simulink model "FinalBidirectionalACDC"  (R2020b)
settings: Solver=VariableStepAuto  StartTime=0.0  StopTime=10.0  RelTol=1e-3
libraries: powerlib x46, powerlib_meascontrol x13, pid_lib x4, eePowerMeasurement x1, simulink x1
settings Model: Creator=Matthew  LastModifiedBy=Matthew

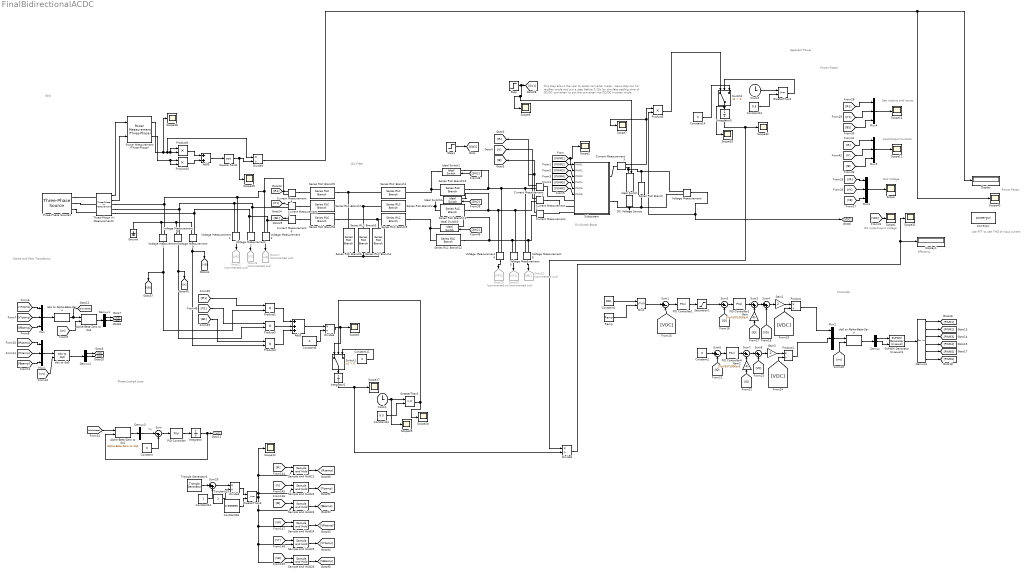
== system FinalBidirectionalACDC ==
  note: Power Factor
  note: Use FFT to see THD of input current
  note: Efficiency
  note: This step allows the user to select converter mode -
      |  leave step low for rectifier mode and put a step before 0.15s
      | (to simulate settling time of DC/DC converter) to put the converter
      | into DC/DC inverter mode.
  note: DC output/input voltage
  note: Power Factor
  note: Apparent Power
  note: Grid
  note: Vq
  note: Phase-Locked
      | Loop
  note: Six-Switch
      | Boost
  note: Grid Voltage
  note: LCL Filter
  note: See outputs and inputs
  note: Input/Output Currents
  note: Clarke and Park
      | Transforms
  note: Controller
  Add3 : Sum  Inputs=+++
  Add6 : Sum
  Alpha-Beta-Zero to dq0 : powerlib_meascontrol/Transformations/Alpha-Beta-Zero to dq0  Alignment=90 degrees behind phase A axis
  Alpha-Beta-Zero to dq1 : powerlib_meascontrol/Transformations/Alpha-Beta-Zero to dq0  Alignment=90 degrees behind phase A axis
  Clock1 : Clock
  Clock2 : Clock
  Constant{,2,11,14} (4 alike) : Constant  Value=0
  Constant1 : Constant  Value=800
  Constant12 : Constant  Value=0.5
  Constant13 : Constant  Value=0.5
  Constant24 : Constant
  Constant25 : Constant  Value=2
  Constant26 : Constant  Value=0.999999
  Constant6 : Constant  Value=-1
  Current Measurement{,1..6} (7 alike) : powerlib/Measurements/Current Measurement  PhasorSimulation=off  OutputType=Complex  PSBequivalent=0
  DC Voltage Source : powerlib/Electrical Sources/DC Voltage Source  Amplitude=800  Measurements=None
  Demux{,1..3} (4 alike) : Demux  Outputs=3
  Demux4 : Demux  Outputs=6
  Display : Display
  Display1 : Display
  Divide{3,6,8..9} (4 alike) : Product  Inputs=*/
  Gain : Gain  Gain=2*pi*50*1000e-6
  Gain1 : Gain  Gain=2
  Gain2 : Gain  Gain=2*pi*50*1000e-6
  Gain3 : Gain  Gain=2
  Goto22 : Goto  Commented=on  GotoTag=VR
  Goto26 : Goto  Commented=on  GotoTag=VY
  Goto27 : Goto  Commented=on  GotoTag=VB
  Goto29 : Goto  Commented=on  GotoTag=VR1
  Goto30 : Goto  Commented=on  GotoTag=VY1
  Goto33 : Goto  Commented=on  GotoTag=VB1
  GreaterThan1 : RelationalOperator  OutDataTypeStr=boolean  RndMeth=Simplest
  GreaterThan2 : RelationalOperator  OutDataTypeStr=boolean  RndMeth=Simplest
  GreaterThan3 : RelationalOperator  OutDataTypeStr=boolean  RndMeth=Simplest
  Ground : powerlib/Elements/Ground  LConnTagsString=a
  Ideal Switch : powerlib/Power Electronics/Ideal Switch  Ron=1e-15  Lon=0  IC=0  Rs=inf  Cs=inf  Measurements=off
  Ideal Switch1 : powerlib/Power Electronics/Ideal Switch  Ron=1e-9  Lon=0  IC=0  Rs=inf  Cs=inf  Measurements=off
  Ideal Switch2 : powerlib/Power Electronics/Ideal Switch  Ron=1e-9  Lon=0  IC=0  Rs=inf  Cs=inf  Measurements=off
  Ideal Switch3 : powerlib/Power Electronics/Ideal Switch  Ron=1e-9  Lon=0  IC=0  Rs=inf  Cs=inf  Measurements=off
  Integrator : Integrator
  Integrator2 : Integrator
  Integrator3 : Integrator
  Min1 : MinMax  Inputs=2
  Mux{,1..5} (6 alike) : Mux  Inputs=3
  PID Controller : pid_lib/PID Controller  Controller=PI  Form=Parallel  TimeDomain=Continuous-time  UseExternalTs=off  SampleTime=-1  IntegratorMethod=Forward Euler  FilterMethod=Forward Euler  ControllerParametersSource=internal  P=10  I=100000  D=0  UseFilter=on  N=100  TunerSelectOption=Transfer Function Based (PID Tuner App)  InitialConditionSource=internal  InitialConditionForIntegrator=0  InitialConditionForFilter=0  DifferentiatorICPrevScaledInput=0  ExternalReset=none  TrackingMode=off  Kt=1  LimitOutput=off  SatLimitsSource=internal  UpperSaturationLimit=inf  LowerSaturationLimit=-inf  LinearizeAsGain=on  AntiWindupMode=none  Kb=1  POutMin=[]  POutMax=[]  IOutMin=[]  IOutMax=[]  DOutMin=[]  DOutMax=[]  NOutMin=[]  NOutMax=[]  SumOutMin=[]  SumOutMax=[]  SaturationOutMin=[]  SaturationOutMax=[]  PParamMin=[]  PParamMax=[]  IParamMin=[]  IParamMax=[]  DParamMin=[]  DParamMax=[]  NParamMin=[]  NParamMax=[]  KbParamMin=[]  KbParamMax=[]  KtParamMin=[]  KtParamMax=[]  KbOutMin=[]  KbOutMax=[]  KtOutMin=[]  KtOutMax=[]  IntegratorOutMin=[]  IntegratorOutMax=[]  FilterOutMin=[]  FilterOutMax=[]  SumI1OutMin=[]  SumI1OutMax=[]  SumI2OutMin=[]  SumI2OutMax=[]  SumI3OutMin=[]  SumI3OutMax=[]  SumI4OutMin=[]  SumI4OutMax=[]  SumDOutMin=[]  SumDOutMax=[]  DifferentiatorOutMin=[]  DifferentiatorOutMax=[]  FilterDiffOutCoefMin=[]  FilterDiffOutCoefMax=[]  ReciprocalOutMin=[]  ReciprocalOutMax=[]  SumDenOutMin=[]  SumDenOutMax=[]  SumNumOutMin=[]  SumNumOutMax=[]  DivideOutMin=[]  DivideOutMax=[]  UdiffTsProdOutMin=[]  UdiffTsProdOutMax=[]  NTsProdOutMin=[]  NTsProdOutMax=[]  UintegralTsProdOutMin=[]  UintegralTsProdOutMax=[]  UngainTsProdOutMin=[]  UngainTsProdOutMax=[]  IntegratorContinuousStateAttributes=''  IntegratorStateMustResolveToSignalObject=off  IntegratorRTWStateStorageClass=Auto  FilterContinuousStateAttributes=''  FilterStateMustResolveToSignalObject=off  FilterRTWStateStorageClass=Auto  ParallelPVariant=InternalParameters  IdealPVariant=Disabled  IVariant=InternalParameters  DVariant=Disabled  IntegratorVariant=Continuous  SatVariant=Disabled  AWVariant=Passthrough  PCopyVariant=Disabled  TRVariant=Disabled  FdbkBlocksVariant=Forward  IdealPFdbkVariant=Disabled  SatFdbkVariant=Disabled  DerivativeFilterVariant=Disabled  NVariant=Disabled  NCopyVariant=Disabled_SignalSpec  FilterICVariant=Disabled  IntegratorICVariant=InternalICs  ExternalResetVariant=Disabled  TRSumVariant=Passthrough  SumFdbkVariant=Disabled  SumVariant=Sum_PI  TsampFilterVariant=InternalTs  TsampNgainVariant=Passthrough  TsampIntegralVariant=Passthrough  ExternalSaturationOutDataTypeStr=Inherit: Same as second input
  PID Controller1 : pid_lib/PID Controller  Controller=PI  Form=Parallel  TimeDomain=Continuous-time  UseExternalTs=off  SampleTime=-1  IntegratorMethod=Forward Euler  FilterMethod=Forward Euler  ControllerParametersSource=internal  P=0.15  I=22  D=0  UseFilter=on  N=100  TunerSelectOption=Transfer Function Based (PID Tuner App)  InitialConditionSource=internal  InitialConditionForIntegrator=0  InitialConditionForFilter=0  DifferentiatorICPrevScaledInput=0  ExternalReset=none  TrackingMode=off  Kt=1  LimitOutput=off  SatLimitsSource=internal  UpperSaturationLimit=inf  LowerSaturationLimit=-inf  LinearizeAsGain=on  AntiWindupMode=none  Kb=1  POutMin=[]  POutMax=[]  IOutMin=[]  IOutMax=[]  DOutMin=[]  DOutMax=[]  NOutMin=[]  NOutMax=[]  SumOutMin=[]  SumOutMax=[]  SaturationOutMin=[]  SaturationOutMax=[]  PParamMin=[]  PParamMax=[]  IParamMin=[]  IParamMax=[]  DParamMin=[]  DParamMax=[]  NParamMin=[]  NParamMax=[]  KbParamMin=[]  KbParamMax=[]  KtParamMin=[]  KtParamMax=[]  KbOutMin=[]  KbOutMax=[]  KtOutMin=[]  KtOutMax=[]  IntegratorOutMin=[]  IntegratorOutMax=[]  FilterOutMin=[]  FilterOutMax=[]  SumI1OutMin=[]  SumI1OutMax=[]  SumI2OutMin=[]  SumI2OutMax=[]  SumI3OutMin=[]  SumI3OutMax=[]  SumI4OutMin=[]  SumI4OutMax=[]  SumDOutMin=[]  SumDOutMax=[]  DifferentiatorOutMin=[]  DifferentiatorOutMax=[]  FilterDiffOutCoefMin=[]  FilterDiffOutCoefMax=[]  ReciprocalOutMin=[]  ReciprocalOutMax=[]  SumDenOutMin=[]  SumDenOutMax=[]  SumNumOutMin=[]  SumNumOutMax=[]  DivideOutMin=[]  DivideOutMax=[]  UdiffTsProdOutMin=[]  UdiffTsProdOutMax=[]  NTsProdOutMin=[]  NTsProdOutMax=[]  UintegralTsProdOutMin=[]  UintegralTsProdOutMax=[]  UngainTsProdOutMin=[]  UngainTsProdOutMax=[]  IntegratorContinuousStateAttributes=''  IntegratorStateMustResolveToSignalObject=off  IntegratorRTWStateStorageClass=Auto  FilterContinuousStateAttributes=''  FilterStateMustResolveToSignalObject=off  FilterRTWStateStorageClass=Auto  ParallelPVariant=InternalParameters  IdealPVariant=Disabled  IVariant=InternalParameters  DVariant=Disabled  IntegratorVariant=Continuous  SatVariant=Disabled  AWVariant=Passthrough  PCopyVariant=Disabled  TRVariant=Disabled  FdbkBlocksVariant=Forward  IdealPFdbkVariant=Disabled  SatFdbkVariant=Disabled  DerivativeFilterVariant=Disabled  NVariant=Disabled  NCopyVariant=Disabled_SignalSpec  FilterICVariant=Disabled  IntegratorICVariant=InternalICs  ExternalResetVariant=Disabled  TRSumVariant=Passthrough  SumFdbkVariant=Disabled  SumVariant=Sum_PI  TsampFilterVariant=InternalTs  TsampNgainVariant=Passthrough  TsampIntegralVariant=Passthrough  ExternalSaturationOutDataTypeStr=Inherit: Same as second input
  PID Controller2 : pid_lib/PID Controller  Controller=PI  Form=Parallel  TimeDomain=Continuous-time  UseExternalTs=off  SampleTime=-1  IntegratorMethod=Forward Euler  FilterMethod=Forward Euler  ControllerParametersSource=internal  P=25  I=500  D=0  UseFilter=on  N=100  TunerSelectOption=Transfer Function Based (PID Tuner App)  InitialConditionSource=internal  InitialConditionForIntegrator=0  InitialConditionForFilter=0  DifferentiatorICPrevScaledInput=0  ExternalReset=none  TrackingMode=off  Kt=1  LimitOutput=off  SatLimitsSource=internal  UpperSaturationLimit=inf  LowerSaturationLimit=-inf  LinearizeAsGain=on  AntiWindupMode=none  Kb=1  POutMin=[]  POutMax=[]  IOutMin=[]  IOutMax=[]  DOutMin=[]  DOutMax=[]  NOutMin=[]  NOutMax=[]  SumOutMin=[]  SumOutMax=[]  SaturationOutMin=[]  SaturationOutMax=[]  PParamMin=[]  PParamMax=[]  IParamMin=[]  IParamMax=[]  DParamMin=[]  DParamMax=[]  NParamMin=[]  NParamMax=[]  KbParamMin=[]  KbParamMax=[]  KtParamMin=[]  KtParamMax=[]  KbOutMin=[]  KbOutMax=[]  KtOutMin=[]  KtOutMax=[]  IntegratorOutMin=[]  IntegratorOutMax=[]  FilterOutMin=[]  FilterOutMax=[]  SumI1OutMin=[]  SumI1OutMax=[]  SumI2OutMin=[]  SumI2OutMax=[]  SumI3OutMin=[]  SumI3OutMax=[]  SumI4OutMin=[]  SumI4OutMax=[]  SumDOutMin=[]  SumDOutMax=[]  DifferentiatorOutMin=[]  DifferentiatorOutMax=[]  FilterDiffOutCoefMin=[]  FilterDiffOutCoefMax=[]  ReciprocalOutMin=[]  ReciprocalOutMax=[]  SumDenOutMin=[]  SumDenOutMax=[]  SumNumOutMin=[]  SumNumOutMax=[]  DivideOutMin=[]  DivideOutMax=[]  UdiffTsProdOutMin=[]  UdiffTsProdOutMax=[]  NTsProdOutMin=[]  NTsProdOutMax=[]  UintegralTsProdOutMin=[]  UintegralTsProdOutMax=[]  UngainTsProdOutMin=[]  UngainTsProdOutMax=[]  IntegratorContinuousStateAttributes=''  IntegratorStateMustResolveToSignalObject=off  IntegratorRTWStateStorageClass=Auto  FilterContinuousStateAttributes=''  FilterStateMustResolveToSignalObject=off  FilterRTWStateStorageClass=Auto  ParallelPVariant=InternalParameters  IdealPVariant=Disabled  IVariant=InternalParameters  DVariant=Disabled  IntegratorVariant=Continuous  SatVariant=Disabled  AWVariant=Passthrough  PCopyVariant=Disabled  TRVariant=Disabled  FdbkBlocksVariant=Forward  IdealPFdbkVariant=Disabled  SatFdbkVariant=Disabled  DerivativeFilterVariant=Disabled  NVariant=Disabled  NCopyVariant=Disabled_SignalSpec  FilterICVariant=Disabled  IntegratorICVariant=InternalICs  ExternalResetVariant=Disabled  TRSumVariant=Passthrough  SumFdbkVariant=Disabled  SumVariant=Sum_PI  TsampFilterVariant=InternalTs  TsampNgainVariant=Passthrough  TsampIntegralVariant=Passthrough  ExternalSaturationOutDataTypeStr=Inherit: Same as second input
  PID Controller4 : pid_lib/PID Controller  Controller=PI  Form=Parallel  TimeDomain=Continuous-time  UseExternalTs=off  SampleTime=-1  IntegratorMethod=Forward Euler  FilterMethod=Forward Euler  ControllerParametersSource=internal  P=25  I=500  D=0  UseFilter=on  N=100  TunerSelectOption=Transfer Function Based (PID Tuner App)  InitialConditionSource=internal  InitialConditionForIntegrator=0  InitialConditionForFilter=0  DifferentiatorICPrevScaledInput=0  ExternalReset=none  TrackingMode=off  Kt=1  LimitOutput=off  SatLimitsSource=internal  UpperSaturationLimit=inf  LowerSaturationLimit=-inf  LinearizeAsGain=on  AntiWindupMode=none  Kb=1  POutMin=[]  POutMax=[]  IOutMin=[]  IOutMax=[]  DOutMin=[]  DOutMax=[]  NOutMin=[]  NOutMax=[]  SumOutMin=[]  SumOutMax=[]  SaturationOutMin=[]  SaturationOutMax=[]  PParamMin=[]  PParamMax=[]  IParamMin=[]  IParamMax=[]  DParamMin=[]  DParamMax=[]  NParamMin=[]  NParamMax=[]  KbParamMin=[]  KbParamMax=[]  KtParamMin=[]  KtParamMax=[]  KbOutMin=[]  KbOutMax=[]  KtOutMin=[]  KtOutMax=[]  IntegratorOutMin=[]  IntegratorOutMax=[]  FilterOutMin=[]  FilterOutMax=[]  SumI1OutMin=[]  SumI1OutMax=[]  SumI2OutMin=[]  SumI2OutMax=[]  SumI3OutMin=[]  SumI3OutMax=[]  SumI4OutMin=[]  SumI4OutMax=[]  SumDOutMin=[]  SumDOutMax=[]  DifferentiatorOutMin=[]  DifferentiatorOutMax=[]  FilterDiffOutCoefMin=[]  FilterDiffOutCoefMax=[]  ReciprocalOutMin=[]  ReciprocalOutMax=[]  SumDenOutMin=[]  SumDenOutMax=[]  SumNumOutMin=[]  SumNumOutMax=[]  DivideOutMin=[]  DivideOutMax=[]  UdiffTsProdOutMin=[]  UdiffTsProdOutMax=[]  NTsProdOutMin=[]  NTsProdOutMax=[]  UintegralTsProdOutMin=[]  UintegralTsProdOutMax=[]  UngainTsProdOutMin=[]  UngainTsProdOutMax=[]  IntegratorContinuousStateAttributes=''  IntegratorStateMustResolveToSignalObject=off  IntegratorRTWStateStorageClass=Auto  FilterContinuousStateAttributes=''  FilterStateMustResolveToSignalObject=off  FilterRTWStateStorageClass=Auto  ParallelPVariant=InternalParameters  IdealPVariant=Disabled  IVariant=InternalParameters  DVariant=Disabled  IntegratorVariant=Continuous  SatVariant=Disabled  AWVariant=Passthrough  PCopyVariant=Disabled  TRVariant=Disabled  FdbkBlocksVariant=Forward  IdealPFdbkVariant=Disabled  SatFdbkVariant=Disabled  DerivativeFilterVariant=Disabled  NVariant=Disabled  NCopyVariant=Disabled_SignalSpec  FilterICVariant=Disabled  IntegratorICVariant=InternalICs  ExternalResetVariant=Disabled  TRSumVariant=Passthrough  SumFdbkVariant=Disabled  SumVariant=Sum_PI  TsampFilterVariant=InternalTs  TsampNgainVariant=Passthrough  TsampIntegralVariant=Passthrough  ExternalSaturationOutDataTypeStr=Inherit: Same as second input
  Power Measurement (Three-Phase) : eePowerMeasurement/Power Measurement (Three-Phase)  LabelModeActiveChoice=Continuous  F=50  K=[1]  Seq=Positive  Ts=0
      settings: SourceProductBaseCode=PS
  Product : Product  Inputs=*/
  Product1 : Product  Inputs=*/
  Product{2..5,9..10} (6 alike) : Product
  Ramp : simulink/Sources/Ramp  slope=450  start=0  InitialOutput=700
  SVPWM Generator (2-Level)1 : powerlib_meascontrol/Pulse & Signal Generators/SVPWM Generator (2-Level)  InputType=alpha-beta components  SwitchingPattern=Pattern #2  Fc=100e3  ParUref=[0.8 -30 50]  Ts=0
      settings: SourceProductBaseCode=PS
  Sample and Hold{21..26} (6 alike) : powerlib_meascontrol/Additional Components/Sample and Hold  ic=0  Ts=0
      settings: SourceProductBaseCode=PS
  Saturation1 : Saturate  UpperLimit=450  LowerLimit=-240
  Scope{,1..2,5,7,9,11..12,14,17,28..29,31..33,40,48..49} (18 alike) : Scope
  Series RLC Branch : powerlib/Elements/Series RLC Branch  LConnTagsString=__new0  RConnTagsString=__new0  BranchType=R  Resistance=6.4  Inductance=1e-3  SetiL0=off  InitialCurrent=0  Capacitance=1e-6  Setx0=off  InitialVoltage=0  Measurements=None
  Series RLC Branch{1..2,5,7..9} (6 alike) : powerlib/Elements/Series RLC Branch  LConnTagsString=__new0  RConnTagsString=__new0  BranchType=RL  Resistance=13.5e-3  Inductance=150e-6  SetiL0=off  InitialCurrent=0  Capacitance=0  Setx0=off  InitialVoltage=0  Measurements=None
  Series RLC Branch10 : powerlib/Elements/Series RLC Branch  LConnTagsString=__new0  RConnTagsString=__new0  BranchType=R  Resistance=1  Inductance=1e-3  SetiL0=off  InitialCurrent=0  Capacitance=1e-6  Setx0=off  InitialVoltage=0  Measurements=None
  Series RLC Branch11 : powerlib/Elements/Series RLC Branch  LConnTagsString=__new0  RConnTagsString=__new0  BranchType=R  Resistance=1  Inductance=1e-3  SetiL0=off  InitialCurrent=0  Capacitance=1e-6  Setx0=off  InitialVoltage=0  Measurements=None
  Series RLC Branch12 : powerlib/Elements/Series RLC Branch  LConnTagsString=__new0  RConnTagsString=__new0  BranchType=R  Resistance=1  Inductance=1e-3  SetiL0=off  InitialCurrent=0  Capacitance=1e-6  Setx0=off  InitialVoltage=0  Measurements=None
  Series RLC Branch3 : powerlib/Elements/Series RLC Branch  LConnTagsString=__new0  RConnTagsString=__new0  BranchType=RC  Resistance=10e-3  Inductance=1e-3  SetiL0=off  InitialCurrent=0  Capacitance=2e-5  Setx0=off  InitialVoltage=0  Measurements=None
  Series RLC Branch4 : powerlib/Elements/Series RLC Branch  LConnTagsString=__new0  RConnTagsString=__new0  BranchType=RC  Resistance=10e-3  Inductance=1e-3  SetiL0=off  InitialCurrent=0  Capacitance=2e-5  Setx0=off  InitialVoltage=0  Measurements=None
  Series RLC Branch6 : powerlib/Elements/Series RLC Branch  LConnTagsString=__new0  RConnTagsString=__new0  BranchType=RC  Resistance=10e-3  Inductance=1e-3  SetiL0=off  InitialCurrent=0  Capacitance=2e-5  Setx0=off  InitialVoltage=0  Measurements=None
  Square Root1 : Sqrt  SaturateOnIntegerOverflow=on
  Step : Step  Time=10  SampleTime=0
  Step1 : Step  Time=0.02  SampleTime=0
  Subsystem : Subsystem
  Sum : Sum  Inputs=|-+
  Sum{1..2,6..7} (4 alike) : Sum  Inputs=|+-
  Sum{3..4,8,29} (4 alike) : Sum  Inputs=|++
  Switch1 : Switch  Criteria=u2 > Threshold
  Switch2 : Switch  Criteria=u2 > Threshold
  Three-Phase V-I Measurement2 : powerlib/Measurements/Three-Phase V-I Measurement  VoltageMeasurement=phase-to-ground  SetLabelV=off  LabelV=Vabc  Vpu=off  VpuLL=off  CurrentMeasurement=yes  SetLabelI=off  LabelI=Iabc  Ipu=off  Pbase=100e6  Vbase=500e3  OutputType=Complex  PhasorSimulation=off  PSBequivalent=0
  Three-Phase Source1 : powerlib/Electrical Sources/Three-Phase Source  InternalConnection=Yg  VoltagePhases=off  Voltage=400  PhaseAngle=0  Voltage_phases=[25e3 25e3 25e3]/sqrt(3)  PhaseAngles_phases=[0 -120 +120]  Frequency=50  NonIdealSource=on  SpecifyImpedance=off  Resistance=0  Inductance=0  ShortCircuitLevel=100e6  BaseVoltage=400  XRratio=7  BusType=swing  Pref=10e3  Qref=0  Prefabc=[10e3, 10e3, 10e3]  Qrefabc=[0, 0, 0]  Qmin=-inf  Qmax=inf
  Triangle Generator3 : powerlib_meascontrol/Pulse & Signal Generators/Triangle Generator  Freq=100e3  Phase=180  Ts=0
  Voltage Measurement{,1..9} (10 alike) : powerlib/Measurements/Voltage Measurement  PhasorSimulation=off  OutputType=Complex  PSBequivalent=0
  abc to Alpha-Beta-Zero : powerlib_meascontrol/Transformations/abc to Alpha-Beta-Zero
  abc to dq0 : powerlib_meascontrol/Transformations/abc to dq0  Alignment=90 degrees behind phase A axis
  dq0 to Alpha-Beta-Zero : powerlib_meascontrol/Transformations/dq0 to Alpha-Beta-Zero  Alignment=90 degrees behind phase A axis
      settings: SourceProductBaseCode=PS
  powergui : powerlib/powergui  Priority=1  SimulationMode=Discrete  SampleTime=1e-6  frequency=60  Iterations=50  frequencyindice=0  Pbase=100e6  ErrMax=1e-4  UnitsV=kV  UnitsW=MW  buscounter=0  FunctionMessages=off  echomessages=off  EnableUseOfTLC=off  CurrentSourceSwitches=off  DisableSnubberDevices=off  DisableRonSwitches=off  DisableVfSwitches=off  DisplayEquations=off  AutomaticDiscreteSolvers=off  SolverType=Tustin/Backward Euler (TBE)  Interpol=off  ExternalGateDelay=off  methode=off  Ts=100  x0status=blocks  SPID=on  SwTol=0  HookPort=off  NonlinearTolerance=1e-4  nMaxIteration=100  ContinueOnMaxIteration=off  RestoreLinks=warning  ResistiveCurrentMeasurement=off  Frange=[0:2:500]  Ylog=off  Xlog=on  ShowGrid=off  save=off  variable=ZData  structure=Current  ZoomFFT=off  StartTime=0.6  cycles=7  DisplayStyle=1  fundamental=50  FreqAxis=off  MaxFrequency=200  frequencyindicesteady=1  RmsSteady=1  display=off
  wires:
  ? -> ?
  Mux4/1 -> Scope14/1
  Min1/1 -> Sum1/1
  Divide6/1 -> Switch1/1, Scope5/1
  [IB1] -> Product4/1
  Ramp/1 -> Min1/2
  Voltage Measurement8/1 -> [VY], Product3/2
  Power Measurement (Three-Phase)/2 -> Product10/2, Product10/1
  Square Root1/1 -> Scope49/1, Divide9/2
  Divide9/1 -> Display/1, Scope40/1
  PID Controller2/1 -> Sum3/1
  Power Measurement (Three-Phase)/1 -> Scope48/1, Divide9/1, Product9/1, Product9/2
  Triangle Generator3/1 -> Sum29/1
  Three-Phase V-I Measurement2/2 -> Power Measurement (Three-Phase)/2
  Alpha-Beta-Zero to dq1/1 -> Demux3/1
  Voltage Measurement3/1 -> Goto27/1
  Current Measurement4/1 -> [IR1]
  Product1/1 -> Mux2/2
  Three-Phase V-I Measurement2/1 -> Power Measurement (Three-Phase)/1
  [VQ] -> Sum8/2
  [VB] -> Mux3/3
  Product9/1 -> Add6/1
  Constant25/1 -> Divide3/2
  [IY] -> Sample and Hold22/1
  Integrator3/1 -> Divide8/1, Scope32/1
  Switch2/1 -> Scope33/1, Integrator3/1
  Current Measurement6/1 -> [IB1]
  Gain3/1 -> Product1/1
  Clock1/1 -> Scope29/1, GreaterThan1/1
  Voltage Measurement7/1 -> [VR], Product2/2
  Add3/1 -> Divide6/1
  Mux5/1 -> Scope11/1
  Switch1/1 -> Integrator2/1
  Constant11/1 -> Switch1/3
  Add6/1 -> Square Root1/1
  [PWM4] -> Subsystem/4(PWM4)
  GreaterThan1/1 -> Switch1/2, Scope28/1
  Divide8/1 -> Scope31/1, Display1/1
  GreaterThan2/1 -> Switch2/2
  abc to Alpha-Beta-Zero/1 -> [alphabeta], Alpha-Beta-Zero to dq0/1
  [IB1] -> Mux4/3
  [VD] -> Sum4/2
  Product5/1 -> Switch2/1
  Constant6/1 -> Divide6/2
  Constant12/1 -> GreaterThan1/2
  Voltage Measurement9/1 -> [VB], Product4/2
  Voltage Measurement5/1 -> Goto30/1
  Product10/1 -> Add6/2
  Sum29/1 -> Divide3/1
  [IB] -> Sample and Hold23/1
  Demux1/2 -> [VQ]
  Integrator2/1 -> Divide8/2, Scope17/1
  dq0 to Alpha-Beta-Zero/1 -> Demux/1
  Demux/1 -> SVPWM Generator (2-Level)1/1
  Demux4/3 -> [PWM3]
  Sum8/1 -> Gain3/1
  [ID] -> Gain2/1
  Mux3/1 -> Scope/1
  Demux4/4 -> [PWM4]
  [VDC] -> Product/2
  [VDC] -> Product1/2
  Demux4/2 -> [PWM2]
  Constant26/1 -> GreaterThan3/2
  Gain1/1 -> Product/1
  Sum4/1 -> Gain1/1
  Sum1/1 -> PID Controller1/1
  [alphabeta] -> Alpha-Beta-Zero to dq1/1
  Integrator/1 -> [wt], Alpha-Beta-Zero to dq1/2
  Sum2/1 -> PID Controller2/1
  [IBsamp] -> Mux1/3
  Sum3/1 -> Sum4/1
  Mux1/1 -> abc to dq0/1
  [IRsamp] -> Mux1/1
  [IQ] -> Gain/1
  Gain/1 -> Sum3/2
  PID Controller/1 -> Integrator/1
  abc to dq0/1 -> Demux2/1
  Demux3/2 -> Sum/1
  Sum/1 -> PID Controller/1
  Current Measurement2/1 -> [IR]
  [wt] -> Alpha-Beta-Zero to dq0/2
  [VBsamp] -> Mux/3
  [PWM3] -> Subsystem/3(PWM3)
  [PWM2] -> Subsystem/2(PWM2)
  Demux2/1 -> [ID]
  Demux1/1 -> [VD]
  [VYsamp] -> Mux/2
  Current Measurement1/1 -> [IY]
  [VDC] -> Sum1/2
  Sum7/1 -> Sum8/1
  Divide3/1 -> GreaterThan3/1
  Saturation1/1 -> Sum2/1
  [IR1] -> Mux4/1
  [VR] -> Mux3/1
  [IB] -> Mux5/3
  Mux2/1 -> dq0 to Alpha-Beta-Zero/1
  [IYsamp] -> Mux1/2
  Step/1 -> Ideal Switch/1, Scope9/1, [Sw1]
  [IR] -> Mux5/1
  [VY] -> Mux3/2
  Voltage Measurement1/1 -> Goto22/1
  Sample and Hold25/1 -> [VYsamp]
  GreaterThan3/1 -> Scope12/1, Sample and Hold21/2, Sample and Hold22/2, Sample and Hold23/2, Sample and Hold24/2, Sample and Hold25/2, Sample and Hold26/2
  Sample and Hold24/1 -> [VRsamp]
  Constant24/1 -> Sum29/2
  [PWM5] -> Subsystem/5(PWM5)
  Sample and Hold26/1 -> [VBsamp]
  Sample and Hold21/1 -> [IRsamp]
  PID Controller4/1 -> Sum7/1
  Sample and Hold22/1 -> [IYsamp]
  [VY] -> Sample and Hold25/1
  [IY1] -> Mux4/2
  [VR] -> Sample and Hold24/1
  Demux4/5 -> [PWM5]
  [IY1] -> Product3/1
  [SW2] -> Ideal Switch3/1
  [SW2] -> Ideal Switch2/1
  Step1/1 -> [SW2]
  Clock2/1 -> GreaterThan2/1
  Current Measurement5/1 -> [IY1]
  [SW2] -> Ideal Switch1/1
  [wt] -> abc to dq0/2
  [ID] -> Sum2/2
  PID Controller1/1 -> Saturation1/1
  [IR] -> Sample and Hold21/1
  [PWM6] -> Subsystem/6(PWM6)
  Constant14/1 -> Switch2/3
  Sum6/1 -> PID Controller4/1
  Sample and Hold23/1 -> [IBsamp]
  Demux2/2 -> [IQ]
  Demux/2 -> SVPWM Generator (2-Level)1/2
  [IY] -> Mux5/2
  Constant1/1 -> Min1/1
  [VDC] -> Scope1/1
  Gain2/1 -> Sum7/2
  Demux4/1 -> [PWM1]
  [VRsamp] -> Mux/1
  Demux4/6 -> [PWM6]
  [VB] -> Sample and Hold26/1
  Constant13/1 -> GreaterThan2/2
  Alpha-Beta-Zero to dq0/1 -> Demux1/1
  SVPWM Generator (2-Level)1/1 -> Demux4/1
  [wt] -> dq0 to Alpha-Beta-Zero/2
  Product2/1 -> Add3/1
  Voltage Measurement6/1 -> Goto33/1
  Voltage Measurement2/1 -> Goto26/1
  Current Measurement3/1 -> Scope7/1, Product5/1
  Constant2/1 -> Sum6/1
  Mux/1 -> abc to Alpha-Beta-Zero/1
  Product/1 -> Mux2/1
  [IR1] -> Product2/1
  Constant/1 -> Sum/2
  Voltage Measurement4/1 -> Goto29/1
  Voltage Measurement/1 -> Product5/2, [VDC]
  Product3/1 -> Add3/2
  [PWM1] -> Scope2/1, Subsystem/1(PWM1)
  Product4/1 -> Add3/3
  [IQ] -> Sum6/2
  Current Measurement/1 -> [IB]
  connections:
  Voltage Measurement8/LConn2 -- Ground/LConn1 -- Voltage Measurement7/LConn2 -- Voltage Measurement9/LConn2
  Series RLC Branch5/LConn1 -- Series RLC Branch6/LConn1 -- Series RLC Branch1/RConn1
  Series RLC Branch/RConn1 -- Subsystem/RConn2 -- DC Voltage Source/LConn1 -- Voltage Measurement/LConn2
  Ideal Switch3/RConn1 -- Series RLC Branch9/LConn1 -- Series RLC Branch12/LConn1
  Voltage Measurement/LConn1 -- Current Measurement3/RConn1 -- Ideal Switch/LConn1 -- Series RLC Branch/LConn1
  Current Measurement2/RConn1 -- Series RLC Branch10/RConn1 -- Ideal Switch1/LConn1 -- Voltage Measurement4/LConn1 -- Voltage Measurement6/LConn2
  Series RLC Branch7/LConn1 -- Series RLC Branch3/LConn1 -- Series RLC Branch2/RConn1
  Series RLC Branch8/LConn1 -- Series RLC Branch4/LConn1 -- Series RLC Branch9/RConn1
  Current Measurement5/RConn1 -- Voltage Measurement2/LConn1 -- Three-Phase V-I Measurement2/RConn2 -- Voltage Measurement8/LConn1 -- Voltage Measurement1/LConn2
  Ideal Switch2/RConn1 -- Series RLC Branch2/LConn1 -- Series RLC Branch11/LConn1
  Series RLC Branch3/RConn1 -- Series RLC Branch6/RConn1 -- Series RLC Branch4/RConn1
  Voltage Measurement7/LConn1 -- Voltage Measurement3/LConn2 -- Current Measurement4/RConn1 -- Voltage Measurement1/LConn1 -- Three-Phase V-I Measurement2/RConn1
  Voltage Measurement9/LConn1 -- Current Measurement6/RConn1 -- Voltage Measurement3/LConn1 -- Voltage Measurement2/LConn2 -- Three-Phase V-I Measurement2/RConn3
  Current Measurement1/RConn1 -- Series RLC Branch11/RConn1 -- Ideal Switch2/LConn1 -- Voltage Measurement4/LConn2 -- Voltage Measurement5/LConn1
  Ideal Switch1/RConn1 -- Series RLC Branch10/LConn1 -- Series RLC Branch1/LConn1
  Current Measurement/RConn1 -- Series RLC Branch12/RConn1 -- Ideal Switch3/LConn1 -- Voltage Measurement5/LConn2 -- Voltage Measurement6/LConn1
  Subsystem/LConn3 -- Current Measurement/LConn1
  Three-Phase Source1/RConn1 -- Three-Phase V-I Measurement2/LConn1
  Subsystem/LConn1 -- Current Measurement2/LConn1
  Current Measurement5/LConn1 -- Series RLC Branch7/RConn1
  Current Measurement1/LConn1 -- Subsystem/LConn2
  Ideal Switch/RConn1 -- DC Voltage Source/RConn1
  Three-Phase Source1/RConn3 -- Three-Phase V-I Measurement2/LConn3
  Current Measurement3/LConn1 -- Subsystem/RConn1
  Current Measurement6/LConn1 -- Series RLC Branch8/RConn1
  Current Measurement4/LConn1 -- Series RLC Branch5/RConn1
  Three-Phase Source1/RConn2 -- Three-Phase V-I Measurement2/LConn2

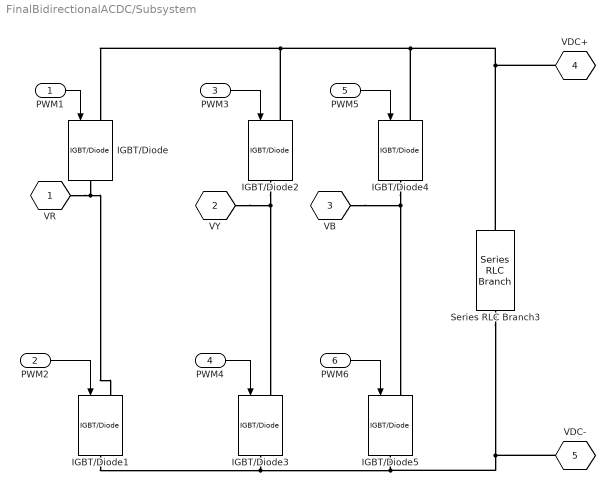
== system FinalBidirectionalACDC/Subsystem ==
  PWM1 : Inport
  PWM2 : Inport  Port=2
  PWM3 : Inport  Port=3
  PWM4 : Inport  Port=4
  PWM5 : Inport  Port=5
  PWM6 : Inport  Port=6
  IGBT/Diode{,1..5} (6 alike) : powerlib/Power Electronics/IGBT//Diode  Ron=1e-3  Rs=1e5  Cs=inf  Measurements=off
  Series RLC Branch3 : powerlib/Elements/Series RLC Branch  LConnTagsString=__new0  RConnTagsString=__new0  BranchType=RC  Resistance=10e-3  Inductance=1e-3  SetiL0=off  InitialCurrent=0  Capacitance=5.6e-3  Setx0=off  InitialVoltage=0  Measurements=None
  VR : PMIOPort  Tag=PMCPort  Side=Left
  VY : PMIOPort  Tag=PMCPort  Port=2  Side=Left
  VB : PMIOPort  Tag=PMCPort  Port=3  Side=Left
  VDC+ : PMIOPort  Tag=PMCPort  Port=4  Side=Right
  VDC- : PMIOPort  Tag=PMCPort  Port=5  Side=Right
  wires:
  PWM2/1 -> IGBT/Diode1/1
  PWM3/1 -> IGBT/Diode2/1
  PWM4/1 -> IGBT/Diode3/1
  PWM6/1 -> IGBT/Diode5/1
  PWM5/1 -> IGBT/Diode4/1
  PWM1/1 -> IGBT/Diode/1
  connections:
  IGBT/Diode4/RConn1 -- VB/RConn1 -- IGBT/Diode5/LConn1
  IGBT/Diode5/RConn1 -- VDC-/RConn1 -- Series RLC Branch3/RConn1 -- IGBT/Diode1/RConn1 -- IGBT/Diode3/RConn1
  IGBT/Diode2/RConn1 -- VY/RConn1 -- IGBT/Diode3/LConn1
  IGBT/Diode/RConn1 -- IGBT/Diode1/LConn1 -- VR/RConn1
  IGBT/Diode2/LConn1 -- IGBT/Diode/LConn1 -- IGBT/Diode4/LConn1 -- Series RLC Branch3/LConn1 -- VDC+/RConn1
